simulink model "ny_finalwork_fzg"  (R2019b)
settings: Solver=FixedStepAuto  StartTime=0.0  StopTime=86400  FixedStep=1  RelTol=1e-3
InitFcn:
  | time = 1:24;
  | radiation = [0	0	0	0	0	84	293	515	715	859	875	875	857	809	581	458	215	56	0	0	0	0	0	0];
  | u = [23.19	9.64	3.39	0	0	3.5	5.5	6	0	0	0	22.61	18.53	0	0	0	0	13.36	18.61	25.42	35.02	22.62	36.74	33.53
  | 23.1	0	0	0	16.9	17.9	19.6	20.7	0	0	0	24.4	24.4	0	0	0	0	53.3	53.3	53.3	53.3	53.3	53.3	40.0
  | 56.1	49.7	44.9	40.4	36.8	34.8	36.2	40.4	0	0	0	129.1	102.9	0	0	0	0	20.9	25.9	41.8	60.4	72.5	76.7	75.7
  | ];
  | E_load = u(1,:);
  | H_load = u(2,:);
  | C_load = u(3,:);
settings Model: Creator=C:\Users\盈乐  LastModifiedBy=C:\Users\盈乐

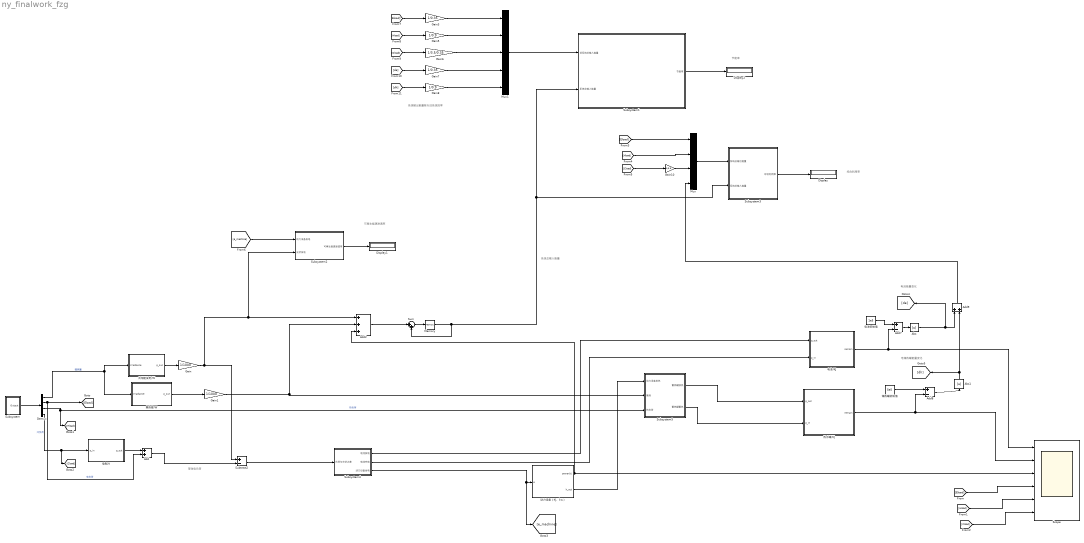
== system ny_finalwork_fzg ==
  note: 系统输出能量除以旧系统效率
  note: 等效电负荷
  note: 节能率
  note: 综合利用率
  note: 可再生能源渗透率
  note: 系统总输入能量
  note: 电池能量变化
  note: 电储热罐能量变化
  Abs : Abs
  Abs1 : Abs
  Add : Sum
  Add2 : Sum  Inputs=+++
  Add7 : Sum  Inputs=+-
  Add8 : Sum  Inputs=+-
  Add9 : Sum
  Demux : Demux
  Display : Display
  Display1 : Display
  Display2 : Display
  Gain : Gain  Gain=1/1000
  Gain1 : Gain  Gain=1/1000
  Gain10 : Gain  Gain=1/3.5
  Gain3 : Gain  Gain=1/0.35
  Gain5 : Gain  Gain=1/0.9
  Gain6 : Gain  Gain=1/3.5/0.35
  Gain7 : Gain  Gain=1/0.35
  Gain8 : Gain  Gain=1/0.9
  Memory : Memory
  Mux : Mux
  Mux1 : Mux  Inputs=5
  Scope : Scope  NumInputPorts=6
  Subsystem : Subsystem
  Subsystem1 : Subsystem
  Subsystem2 : Subsystem
  Subsystem3 : Subsystem
  Subsystem4 : Subsystem
  Subsystem5 : Subsystem
  Subtract2 : Sum  Inputs=+-
  Sum : Sum  Inputs=|++
  储热罐初始值 : Constant  Value=5e5
  动力设备（KJ、kw） : Subsystem  mask{capacity=20, e_hremain=0.7}
      mask Display: image(imread('C:\Users\盈乐\Downloads\pictures\149680720\发动机.jpg'))
  太阳能发电/W : Subsystem  mask{area=100, efficiency=0.17}
      mask prompts: area "area of photovoltaic panel"
      mask Display: image(imread('C:\Users\盈乐\Downloads\pictures\35835164\太阳能电池板和风力涡轮机.jpg'))
  热水罐/KJ : Subsystem  mask{capacity=1e6}
      mask Display: image(imread('C:\Users\盈乐\Downloads\pictures\25136086\孤立的绿瓶.jpg'))
  电制冷 : Subsystem  mask{cop=1/3.5}
      mask prompts: cop "1/cop"
      mask Display: image(imread('C:\Users\盈乐\Downloads\pictures\109413970\家里墙上的空调.jpg'))
  电池/KJ : Subsystem  mask{capacity=2e5, e_in=0.9, e_out=0.9}
      mask prompts: e_in "efficiency for in"; e_out "efficiency for out"
      mask Display: image(imread('C:\Users\盈乐\Downloads\pictures\111398286\电池充满电.jpg'))
  电池初始值 : Constant  Value=1e5
  集热器/W : Subsystem  mask{area=100, efficiency=0.6}
      mask prompts: area "area of photovoltaic panel"
      mask Display: image(imread('C:\Users\盈乐\Downloads\pictures\38491865\工业屋顶上的太阳能电池板.jpg'))
  wires:
  Demux/1 -> 太阳能发电/W/1("irradiance "), 集热器/W/1("irradiance ")  "辐照量"
  集热器/W/1(p_sun) -> Gain1/1
  太阳能发电/W/1(p_sun) -> Gain/1
  Subsystem/1(Output) -> Demux/1
  Demux/2 -> [Eload], Add/2  "电负荷"
  Gain/1 -> Subsystem2/2(光伏发电), Add2/1, Subtract2/1
  Demux/4 -> 电制冷/1(p_in), [Cload]  "冷负荷"
  电制冷/1(p_out) -> Add/1
  Demux/3 -> [Hload], Subsystem5/3(热负荷)  "热负荷"
  Gain1/1 -> Subsystem5/2(集热), Add2/2
  电池/KJ/1(remain) -> Add7/2, Scope/1
  热水罐/KJ/1(remain) -> Add8/2, Scope/2
  [Eload] -> Scope/4
  [Hload] -> Scope/5
  [Cload] -> Scope/6
  动力设备（KJ、kw）/1(power/kJ) -> Scope/3, Add2/3
  Sum/1 -> Memory/1
  Add2/1 -> Sum/1
  [Cload] -> Gain6/1
  电池初始值/1 -> Add7/1
  储热罐初始值/1 -> Add8/1
  Add7/1 -> Abs/1
  Add8/1 -> Abs1/1
  Abs/1 -> Add9/1, [de]
  Abs1/1 -> Add9/2, [dh]
  [Eload] -> Gain3/1
  [Hload] -> Gain5/1
  Add/1 -> Subtract2/2
  [e_machine] -> Subsystem2/1(动力设备发电)
  Subsystem2/1(可再生能源渗透率) -> Display1/1
  [Cload] -> Gain10/1
  Subsystem3/1(综合利用率) -> Display/1
  [Eload] -> Mux/1
  [Hload] -> Mux/2
  Gain10/1 -> Mux/3
  Add9/1 -> Mux/4
  Mux/1 -> Subsystem3/1(系统总输出能量)
  Subsystem4/3(动力设备发电) -> [e_machine], 动力设备（KJ、kw）/1(e)
  Subtract2/1 -> Subsystem4/1(负荷与光伏之差)
  Subsystem4/1(电池放电) -> 电池/KJ/1(p_out)
  Subsystem4/2(电池充电) -> 电池/KJ/2(p_in)
  Subsystem5/1(蓄热罐放热) -> 热水罐/KJ/1(p_out)
  Subsystem5/2(蓄热罐蓄热) -> 热水罐/KJ/2(p_in)
  动力设备（KJ、kw）/2(h_out) -> Subsystem5/1(动力设备发热)
  Gain3/1 -> Mux1/1
  Gain5/1 -> Mux1/2
  Gain6/1 -> Mux1/3
  [dh] -> Gain8/1
  [de] -> Gain7/1
  Memory/1 -> Subsystem3/2(系统总输入能量), Subsystem1/2(系统总输入能量), Sum/2
  Mux1/1 -> Subsystem1/1(旧系统总输入能量)
  Subsystem1/1(节能率) -> Display2/1
  Gain7/1 -> Mux1/4
  Gain8/1 -> Mux1/5

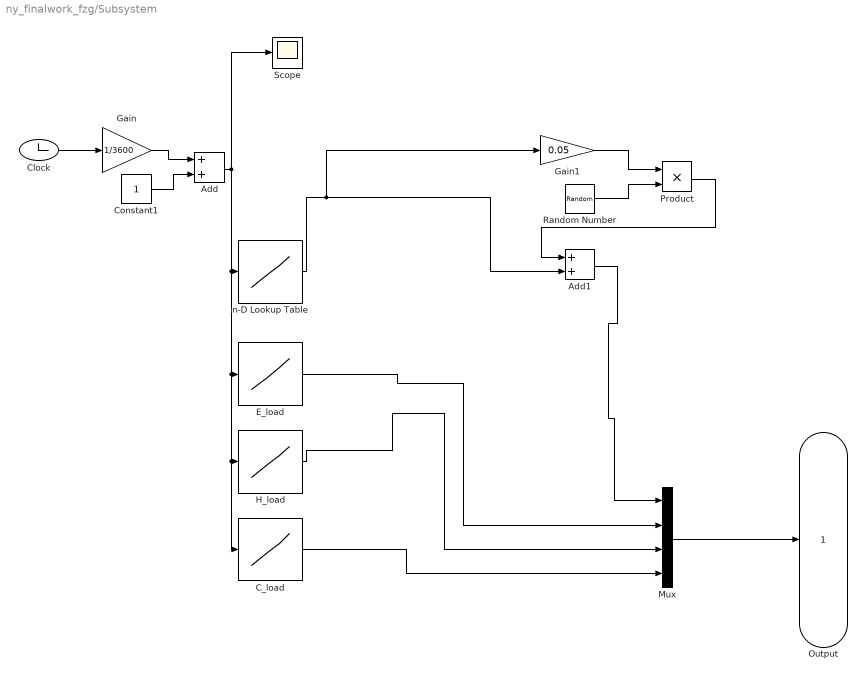
== system ny_finalwork_fzg/Subsystem ==
  Add : Sum
  Add1 : Sum
  C_load : Lookup_n-D  NumberOfTableDimensions=1  BreakpointsForDimension1=time  BreakpointsForDimension3=[5, 7]  Table=C_load  InternalRulePriority=Speed  RndMeth=Simplest  InputSameDT=on
  Clock : Clock
  Constant1 : Constant
  E_load : Lookup_n-D  NumberOfTableDimensions=1  BreakpointsForDimension1=time  BreakpointsForDimension3=[5, 7]  Table=E_load  InternalRulePriority=Speed  RndMeth=Simplest  InputSameDT=on
  Gain : Gain  Gain=1/3600
  Gain1 : Gain  Gain=0.05
  H_load : Lookup_n-D  NumberOfTableDimensions=1  BreakpointsForDimension1=time  BreakpointsForDimension3=[5, 7]  Table=H_load  InternalRulePriority=Speed  RndMeth=Simplest  InputSameDT=on
  Mux : Mux
  Product : Product
  Random Number : RandomNumber  SampleTime=60
  Scope : Scope
  n-D Lookup Table : Lookup_n-D  NumberOfTableDimensions=1  BreakpointsForDimension1=time  BreakpointsForDimension3=[5, 7]  Table=radiation  InternalRulePriority=Speed  RndMeth=Simplest  InputSameDT=on
  Output : Outport
  wires:
  n-D Lookup Table/1 -> Add1/2, Gain1/1
  Gain/1 -> Add/1
  Mux/1 -> Output/1
  Add/1 -> C_load/1, H_load/1, E_load/1, n-D Lookup Table/1, Scope/1
  C_load/1 -> Mux/4
  Clock/1 -> Gain/1
  E_load/1 -> Mux/2
  H_load/1 -> Mux/3
  Constant1/1 -> Add/2
  Add1/1 -> Mux/1
  Gain1/1 -> Product/1
  Product/1 -> Add1/1
  Random Number/1 -> Product/2

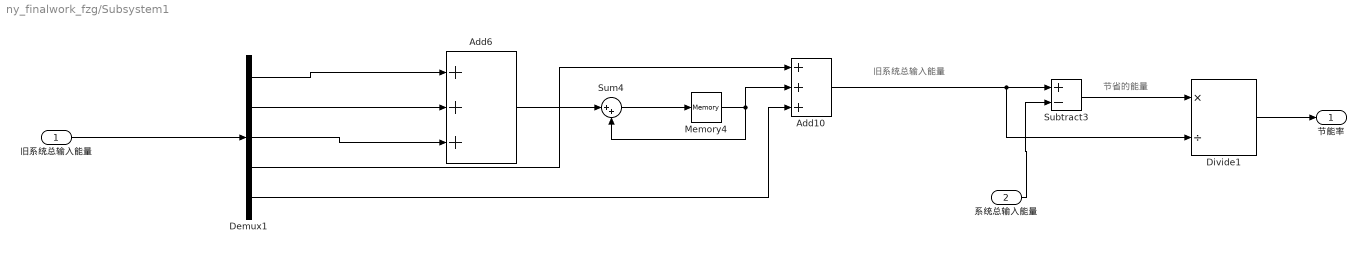
== system ny_finalwork_fzg/Subsystem1 ==
  note: 节省的能量
  note: 旧系统总输入能量
  旧系统总输入能量 : Inport
  系统总输入能量 : Inport  Port=2
  Add10 : Sum  Inputs=+++
  Add6 : Sum  Inputs=+++
  Demux1 : Demux  Outputs=5
  Divide1 : Product  Inputs=*/
  Memory4 : Memory
  Subtract3 : Sum  Inputs=+-
  Sum4 : Sum  Inputs=|++
  节能率 : Outport
  wires:
  Add6/1 -> Sum4/1
  Demux1/2 -> Add6/2
  Subtract3/1 -> Divide1/1
  Sum4/1 -> Memory4/1
  Demux1/3 -> Add6/3
  Memory4/1 -> Sum4/2, Add10/2
  Demux1/1 -> Add6/1
  Add10/1 -> Subtract3/1, Divide1/2
  Divide1/1 -> 节能率/1
  旧系统总输入能量/1 -> Demux1/1
  系统总输入能量/1 -> Subtract3/2
  Demux1/4 -> Add10/1
  Demux1/5 -> Add10/3

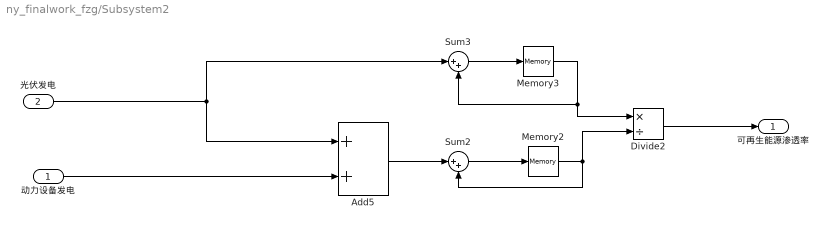
== system ny_finalwork_fzg/Subsystem2 ==
  动力设备发电 : Inport
  光伏发电 : Inport  Port=2
  Add5 : Sum
  Divide2 : Product  Inputs=*/
  Memory2 : Memory
  Memory3 : Memory
  Sum2 : Sum  Inputs=|++
  Sum3 : Sum  Inputs=|++
  可再生能源渗透率 : Outport
  wires:
  动力设备发电/1 -> Add5/2
  Divide2/1 -> 可再生能源渗透率/1
  Add5/1 -> Sum2/1
  Memory2/1 -> Sum2/2, Divide2/2
  Sum3/1 -> Memory3/1
  Memory3/1 -> Divide2/1, Sum3/2
  光伏发电/1 -> Sum3/1, Add5/1
  Sum2/1 -> Memory2/1

== system ny_finalwork_fzg/Subsystem3 ==
  note: 系统总输出能量
  系统总输出能量 : Inport
  系统总输入能量 : Inport  Port=2
  Add3 : Sum  Inputs=+++
  Add4 : Sum
  Demux : Demux
  Divide : Product  Inputs=*/
  Memory1 : Memory
  Sum1 : Sum  Inputs=|++
  综合利用率 : Outport
  wires:
  Add4/1 -> Divide/1
  Memory1/1 -> Sum1/2, Add4/1
  Add3/1 -> Sum1/1
  Divide/1 -> 综合利用率/1
  Sum1/1 -> Memory1/1
  系统总输出能量/1 -> Demux/1
  Demux/1 -> Add3/1
  Demux/2 -> Add3/2
  Demux/3 -> Add3/3
  Demux/4 -> Add4/2
  系统总输入能量/1 -> Divide/2

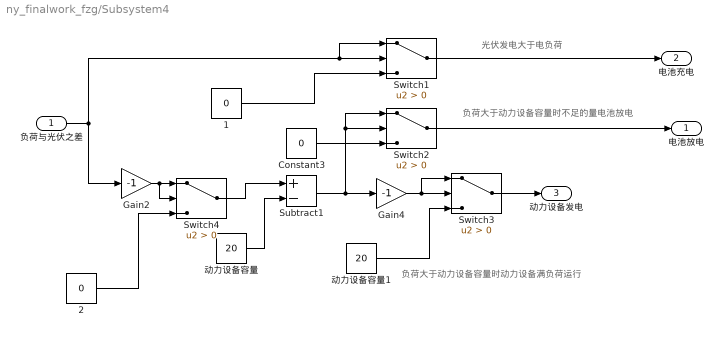
== system ny_finalwork_fzg/Subsystem4 ==
  note: 负荷大于动力设备容量时不足的量电池放电
  note: 光伏发电大于电负荷
  note: 负荷大于动力设备容量时动力设备满负荷运行
  负荷与光伏之差 : Inport
  1 : Constant  Value=0
  2 : Constant  Value=0
  Constant3 : Constant  Value=0
  Gain2 : Gain  Gain=-1
  Gain4 : Gain  Gain=-1
  Subtract1 : Sum  Inputs=+-
  Switch{1..4} (4 alike) : Switch  Criteria=u2 > Threshold
  动力设备容量 : Constant  Value=20
  动力设备容量1 : Constant  Value=20
  电池放电 : Outport
  电池充电 : Outport  Port=2
  动力设备发电 : Outport  Port=3
  wires:
  Gain2/1 -> Switch4/2, Switch4/1
  1/1 -> Switch1/3
  Gain4/1 -> Switch3/1, Switch3/2
  Switch2/1 -> 电池放电/1
  Subtract1/1 -> Gain4/1, Switch2/1, Switch2/2
  动力设备容量1/1 -> Switch3/3
  Switch4/1 -> Subtract1/1
  负荷与光伏之差/1 -> Gain2/1, Switch1/1, Switch1/2
  Constant3/1 -> Switch2/3
  动力设备容量/1 -> Subtract1/2
  2/1 -> Switch4/3
  Switch3/1 -> 动力设备发电/1
  Switch1/1 -> 电池充电/1

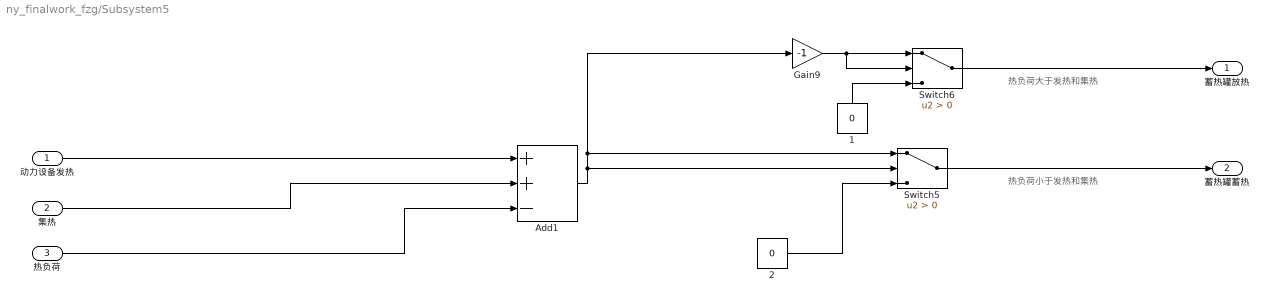
== system ny_finalwork_fzg/Subsystem5 ==
  note: 热负荷小于发热和集热
  note: 热负荷大于发热和集热
  动力设备发热 : Inport
  集热 : Inport  Port=2
  热负荷 : Inport  Port=3
  1 : Constant  Value=0
  2 : Constant  Value=0
  Add1 : Sum  Inputs=++-
  Gain9 : Gain  Gain=-1
  Switch5 : Switch  Criteria=u2 > Threshold
  Switch6 : Switch  Criteria=u2 > Threshold
  蓄热罐放热 : Outport
  蓄热罐蓄热 : Outport  Port=2
  wires:
  Gain9/1 -> Switch6/2, Switch6/1
  Add1/1 -> Switch5/1, Gain9/1, Switch5/2
  1/1 -> Switch6/3
  Switch6/1 -> 蓄热罐放热/1
  2/1 -> Switch5/3
  动力设备发热/1 -> Add1/1
  Switch5/1 -> 蓄热罐蓄热/1
  集热/1 -> Add1/2
  热负荷/1 -> Add1/3

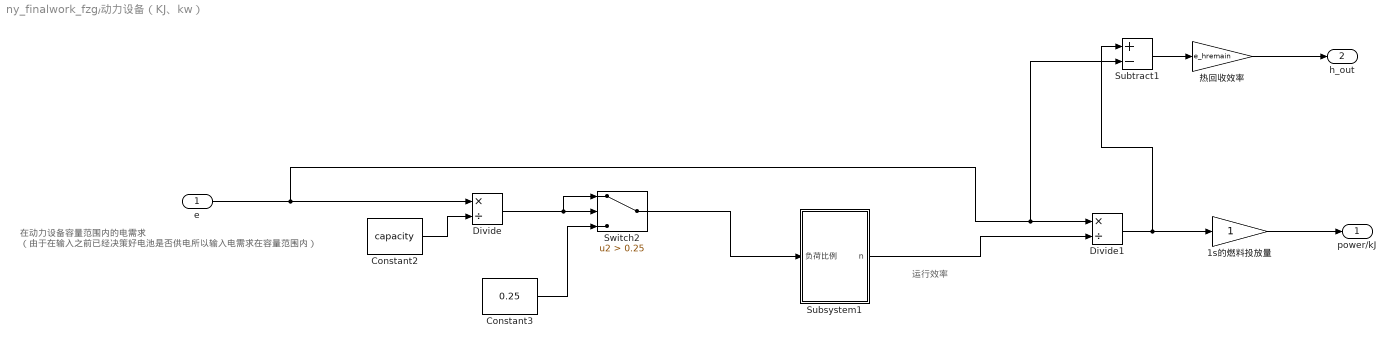
== system ny_finalwork_fzg/动力设备（KJ、kw） ==
  note: 运行效率
  note: 在动力设备容量范围内的电需求
      | （由于在输入之前已经决策好电池是否供电所以输入电需求在容量范围内）
  e : Inport
  1s的燃料投放量 : Gain
  Constant2 : Constant  Value=capacity
  Constant3 : Constant  Value=0.25
  Divide : Product  Inputs=*/
  Divide1 : Product  Inputs=*/
  Subsystem1 : Subsystem
  Subtract1 : Sum  Inputs=+-
  Switch2 : Switch  Criteria=u2 > Threshold  Threshold=0.25
  热回收效率 : Gain  Gain=e_hremain
  power/kJ : Outport
  h_out : Outport  Port=2
  wires:
  Subtract1/1 -> 热回收效率/1
  热回收效率/1 -> h_out/1
  Subsystem1/1(n) -> Divide1/2
  Switch2/1 -> Subsystem1/1(负荷比例)
  Divide/1 -> Switch2/1, Switch2/2
  Divide1/1 -> Subtract1/1, 1s的燃料投放量/1
  Constant2/1 -> Divide/2
  e/1 -> Subtract1/2, Divide1/1, Divide/1
  1s的燃料投放量/1 -> power/kJ/1
  Constant3/1 -> Switch2/3

== system ny_finalwork_fzg/太阳能发电//W ==
  "irradiance " : Inport
  Constant : Constant  Value=area
  Gain : Gain  Gain=efficiency
  Product : Product
  p_sun : Outport
  wires:
  "irradiance "/1 -> Product/1
  Product/1 -> Gain/1
  Gain/1 -> p_sun/1
  Constant/1 -> Product/2

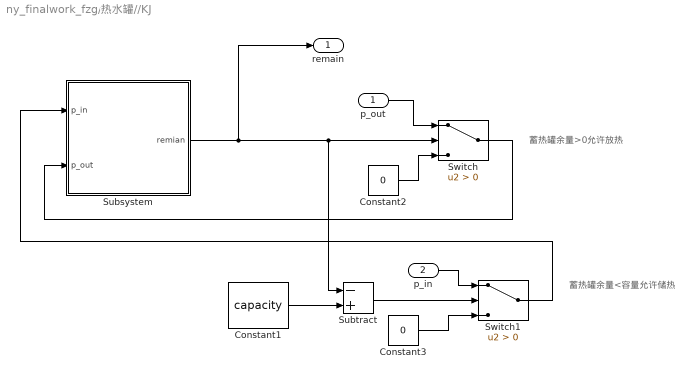
== system ny_finalwork_fzg/热水罐//KJ ==
  note: 蓄热罐余量>0允许放热
  note: 蓄热罐余量<容量允许储热
  p_out : Inport
  p_in : Inport  Port=2
  Constant1 : Constant  Value=capacity
  Constant2 : Constant  Value=0
  Constant3 : Constant  Value=0
  Subsystem : Subsystem
  Subtract : Sum  Inputs=-+
  Switch : Switch  Criteria=u2 > Threshold
  Switch1 : Switch  Criteria=u2 > Threshold
  remain : Outport  VectorParamsAs1DForOutWhenUnconnected=off
  wires:
  Subsystem/1(remian) -> Subtract/1, Switch/2, remain/1
  p_out/1 -> Switch/1
  Constant2/1 -> Switch/3
  Switch/1 -> Subsystem/2(p_out)
  Constant1/1 -> Subtract/2
  Subtract/1 -> Switch1/2
  p_in/1 -> Switch1/1
  Constant3/1 -> Switch1/3
  Switch1/1 -> Subsystem/1(p_in)

== system ny_finalwork_fzg/电制冷 ==
  p_in : Inport
  Multiply : Gain  Gain=cop
  p_out : Outport
  wires:
  p_in/1 -> Multiply/1
  Multiply/1 -> p_out/1

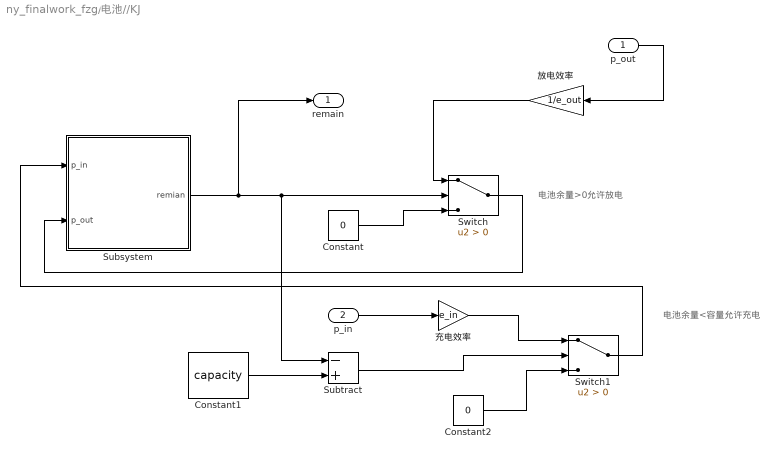
== system ny_finalwork_fzg/电池//KJ ==
  note: 电池余量>0允许放电
  note: 电池余量<容量允许充电
  p_out : Inport
  p_in : Inport  Port=2
  Constant : Constant  Value=0
  Constant1 : Constant  Value=capacity
  Constant2 : Constant  Value=0
  Subsystem : Subsystem
  Subtract : Sum  Inputs=-+
  Switch : Switch  Criteria=u2 > Threshold
  Switch1 : Switch  Criteria=u2 > Threshold
  充电效率 : Gain  Gain=e_in
  放电效率 : Gain  Gain=1/e_out
  remain : Outport  VectorParamsAs1DForOutWhenUnconnected=off
  wires:
  p_out/1 -> 放电效率/1
  Subsystem/1(remian) -> Subtract/1, Switch/2, remain/1
  p_in/1 -> 充电效率/1
  Constant/1 -> Switch/3
  放电效率/1 -> Switch/1
  Switch/1 -> Subsystem/2(p_out)
  Constant1/1 -> Subtract/2
  充电效率/1 -> Switch1/1
  Subtract/1 -> Switch1/2
  Constant2/1 -> Switch1/3
  Switch1/1 -> Subsystem/1(p_in)

== system ny_finalwork_fzg/集热器//W ==
  "irradiance " : Inport
  Constant : Constant  Value=area
  Gain : Gain  Gain=efficiency
  Product : Product
  p_sun : Outport
  wires:
  Constant/1 -> Product/2
  Gain/1 -> p_sun/1
  Product/1 -> Gain/1
  "irradiance "/1 -> Product/1

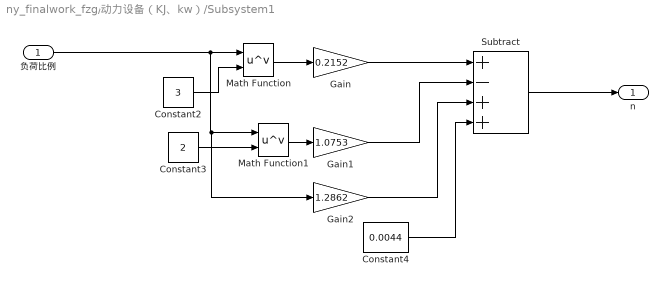
== system ny_finalwork_fzg/动力设备（KJ、kw）/Subsystem1 ==
  负荷比例 : Inport
  Constant2 : Constant  Value=3
  Constant3 : Constant  Value=2
  Constant4 : Constant  Value=0.0044
  Gain : Gain  Gain=0.2152
  Gain1 : Gain  Gain=1.0753
  Gain2 : Gain  Gain=1.2862
  Math Function : Math  Operator=pow  SignedPower=off  SaturateOnIntegerOverflow=on
  Math Function1 : Math  Operator=pow  SignedPower=off  SaturateOnIntegerOverflow=on
  Subtract : Sum  Inputs=+-++
  n : Outport
  wires:
  Constant3/1 -> Math Function1/2
  Math Function/1 -> Gain/1
  Math Function1/1 -> Gain1/1
  Gain2/1 -> Subtract/3
  Gain1/1 -> Subtract/2
  Gain/1 -> Subtract/1
  Constant4/1 -> Subtract/4
  Subtract/1 -> n/1
  Constant2/1 -> Math Function/2
  负荷比例/1 -> Gain2/1, Math Function1/1, Math Function/1

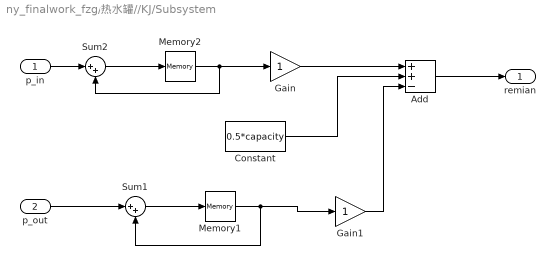
== system ny_finalwork_fzg/热水罐//KJ/Subsystem ==
  p_in : Inport
  p_out : Inport  Port=2
  Add : Sum  Inputs=++-
  Constant : Constant  Value=0.5*capacity
  Gain : Gain
  Gain1 : Gain
  Memory1 : Memory
  Memory2 : Memory
  Sum1 : Sum  Inputs=|++
  Sum2 : Sum  Inputs=|++
  remian : Outport  VectorParamsAs1DForOutWhenUnconnected=off
  wires:
  Gain1/1 -> Add/3
  Gain/1 -> Add/1
  Constant/1 -> Add/2
  p_in/1 -> Sum2/1
  Add/1 -> remian/1
  Sum2/1 -> Memory2/1
  Memory2/1 -> Sum2/2, Gain/1
  Sum1/1 -> Memory1/1
  Memory1/1 -> Sum1/2, Gain1/1
  p_out/1 -> Sum1/1

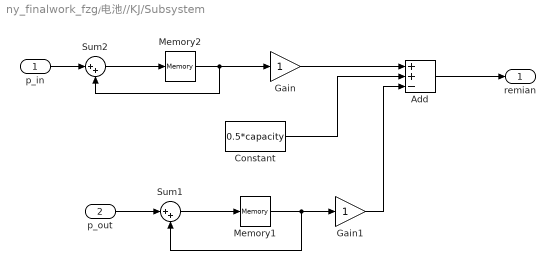
== system ny_finalwork_fzg/电池//KJ/Subsystem ==
  p_in : Inport
  p_out : Inport  Port=2
  Add : Sum  Inputs=++-
  Constant : Constant  Value=0.5*capacity
  Gain : Gain
  Gain1 : Gain
  Memory1 : Memory
  Memory2 : Memory
  Sum1 : Sum  Inputs=|++
  Sum2 : Sum  Inputs=|++
  remian : Outport  VectorParamsAs1DForOutWhenUnconnected=off
  wires:
  Add/1 -> remian/1
  p_in/1 -> Sum2/1
  p_out/1 -> Sum1/1
  Constant/1 -> Add/2
  Gain/1 -> Add/1
  Gain1/1 -> Add/3
  Sum2/1 -> Memory2/1
  Memory2/1 -> Sum2/2, Gain/1
  Sum1/1 -> Memory1/1
  Memory1/1 -> Sum1/2, Gain1/1
